simulink model "smc_ct"  (R2020a)
settings: Solver=FixedStepAuto  StartTime=0.0  StopTime=tstop  FixedStep=tstep  RelTol=1e-3
values from neighbouring files (symbols this model uses):
  Ts = 0.01    [data.m]
  xic = [-2; 1]    [data.m]
  xmic = [-3; -2]    [data.m]
settings Model: Creator=Maithili Shetty  LastModifiedBy=Maithili Shetty
settings DataIOCC: ReturnWorkspaceOutputs=off

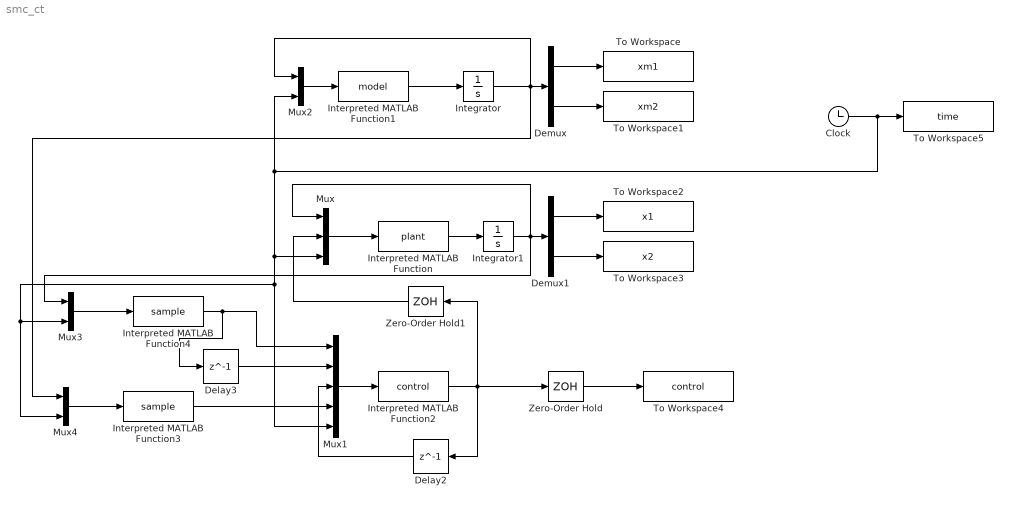
== system smc_ct ==
  Clock : Clock
  Delay2 : Delay  DelayLength=1  SampleTime=Ts
  Delay3 : Delay  DelayLength=1  SampleTime=Ts
  Demux : Demux  Outputs=2
  Demux1 : Demux  Outputs=2
  Integrator : Integrator  InitialCondition=xmic
  Integrator1 : Integrator  InitialCondition=xic
  Interpreted MATLAB Function : MATLABFcn  MATLABFcn=plant  OutputDimensions=2
  Interpreted MATLAB Function1 : MATLABFcn  MATLABFcn=model  OutputDimensions=2
  Interpreted MATLAB Function2 : MATLABFcn  MATLABFcn=control  OutputDimensions=1
  Interpreted MATLAB Function3 : MATLABFcn  MATLABFcn=sample  OutputDimensions=2
  Interpreted MATLAB Function4 : MATLABFcn  MATLABFcn=sample  OutputDimensions=2
  Mux : Mux  Inputs=3
  Mux1 : Mux  Inputs=5
  Mux2 : Mux  Inputs=2
  Mux3 : Mux  Inputs=2
  Mux4 : Mux  Inputs=2
  To Workspace : ToWorkspace  VariableName=xm1  SampleTime=-1
  To Workspace1 : ToWorkspace  VariableName=xm2  SampleTime=-1
  To Workspace2 : ToWorkspace  VariableName=x1  SampleTime=-1
  To Workspace3 : ToWorkspace  VariableName=x2  SampleTime=-1
  To Workspace4 : ToWorkspace  VariableName=control  SampleTime=-1
  To Workspace5 : ToWorkspace  VariableName=time  SampleTime=-1
  Zero-Order Hold : ZeroOrderHold  SampleTime=Ts
  Zero-Order Hold1 : ZeroOrderHold  SampleTime=Ts
  wires:
  Mux2/1 -> Interpreted MATLAB Function1/1
  Delay2/1 -> Mux1/3
  Delay3/1 -> Mux1/2
  Interpreted MATLAB Function2/1 -> Zero-Order Hold1/1, Zero-Order Hold/1, Delay2/1
  Integrator1/1 -> Mux3/1, Mux/1, Demux1/1
  Mux1/1 -> Interpreted MATLAB Function2/1
  Clock/1 -> Mux1/5, Mux4/2, Mux3/2, Mux/3, Mux2/2, To Workspace5/1
  Demux1/1 -> To Workspace2/1
  Demux/1 -> To Workspace/1
  Demux1/2 -> To Workspace3/1
  Mux/1 -> Interpreted MATLAB Function/1
  Interpreted MATLAB Function/1 -> Integrator1/1
  Integrator/1 -> Mux4/1, Mux2/1, Demux/1
  Demux/2 -> To Workspace1/1
  Interpreted MATLAB Function1/1 -> Integrator/1
  Zero-Order Hold/1 -> To Workspace4/1
  Zero-Order Hold1/1 -> Mux/2
  Interpreted MATLAB Function3/1 -> Mux1/4
  Interpreted MATLAB Function4/1 -> Delay3/1, Mux1/1
  Mux3/1 -> Interpreted MATLAB Function4/1
  Mux4/1 -> Interpreted MATLAB Function3/1
